simulink model "dasd"  (R2023a)
settings: Solver=VariableStepAuto  StartTime=0.0  StopTime=10.0  RelTol=1e-3
libraries: simulink x2, commdigbbndpm3 x2, commchan3 x1, commrandsrc3 x1, commsink2 x1
settings Model: Creator=aedan  LastModifiedBy=aedan

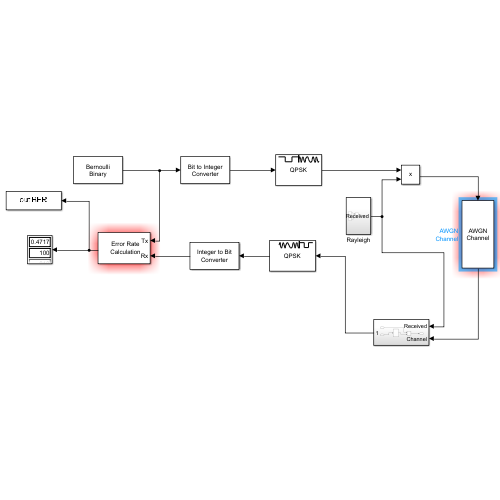
[thumbnail: Simulink's stored preview of the top-level diagram]
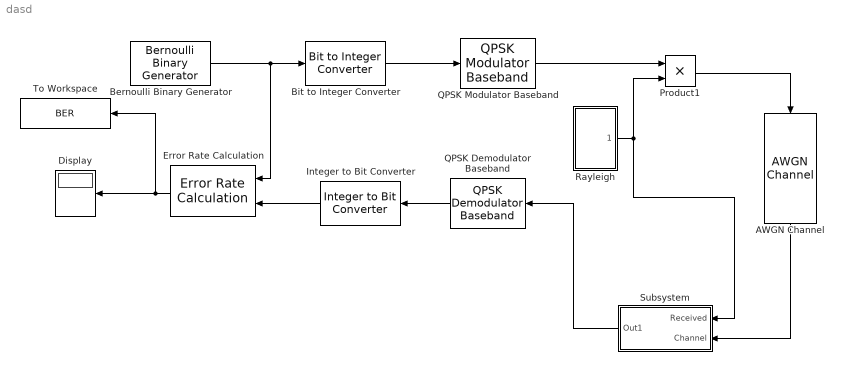
== system dasd ==
  AWGN Channel : commchan3/AWGN Channel  LegacyMode=off  NoiseMethod="Signal to noise ratio  (SNR)"  noiseMode="Signal to noise ratio  (SNR)"  EbNo=EbNo  EsNo=10  SNR=EbNo  BitsPerSymbol=1  SignalPower=1  SamplesPerSymbol=1  SymbolPeriod=1  VarianceSource=Parameter  Variance=1  RandomStream=Global stream  Seed=67  SimulateUsing=Code generation
  Bernoulli Binary Generator : commrandsrc3/Bernoulli Binary Generator  ProbabilityOfZero=0.5  SeedSource=Auto  Seed=0  SampleTime=1e-6  SamplesPerFrame=2  OutputDataType=uint8  SimulateUsing=Interpreted execution
  Bit to Integer Converter : simulink/Logic and Bit Operations/Bit to Integer Converter  nbits=2  bitOrder=MSB first  signedOutputValues=Unsigned  outDtype=Inherit via internal rule  outDtypeSigned=Inherit via internal rule
  Display : Display
  Error Rate Calculation : commsink2/Error Rate Calculation  N=0  st_delay=0  cp_mode=Entire frame  subframe=[]  PMode=Port  WsName=grayBER  RsMode2=off  stop=on  numErr=maxNumErrs  maxBits=maxNumBits
  Integer to Bit Converter : simulink/Logic and Bit Operations/Integer to Bit Converter  nbits=2  signedInputValues=Unsigned  bitOrder=MSB first  outDtype=Inherit via internal rule
      settings: LibrarySourceBlock=|
      | commutil2/Integer to Bit
      | Converter
  Product1 : Product
  QPSK Demodulator Baseband : commdigbbndpm3/QPSK Demodulator Baseband  OutType=Integer  DecType=Hard decision  VarSource=Dialog  Variance=1  Dec=Gray  Ph=pi/4  outDtype1=Inherit via internal rule  outDtype2=Inherit via internal rule  derotateFactorWordLen=16  derotateFactorDataTypeStr=Inherit: Same word length as input  derotateFactorLastDataTypeStr=Inherit: Same word length as input
      settings: LibrarySourceBlock=|
      | commhdldigbbndpm/QPSK
      | Demodulator
      | Baseband
  QPSK Modulator Baseband : commdigbbndpm3/QPSK Modulator Baseband  InType=Integer  Enc=Gray  Ph=pi/4  outDtype=double  outWordLen=16  outUDDataType=sfix(16)  outFracLenMode=Best precision  outFracLen=15  outDataTypeStr=double  outLastDataTypeStr=double
  Rayleigh : Subsystem
  Subsystem : Subsystem
  To Workspace : ToWorkspace  VariableName=BER  SampleTime=-1
      settings: MaxDataPoints=1
  wires:
  Bernoulli Binary Generator/1 -> Error Rate Calculation/1, Bit to Integer Converter/1
  Bit to Integer Converter/1 -> QPSK Modulator Baseband/1
  Integer to Bit Converter/1 -> Error Rate Calculation/2
  QPSK Modulator Baseband/1 -> Product1/1
  Product1/1 -> AWGN Channel/1
  QPSK Demodulator Baseband/1 -> Integer to Bit Converter/1
  Rayleigh/1(Received) -> Subsystem/1(Received), Product1/2
  AWGN Channel/1 -> Subsystem/2(Channel)
  Subsystem/1(Out1) -> QPSK Demodulator Baseband/1
  Error Rate Calculation/1 -> To Workspace/1, Display/1

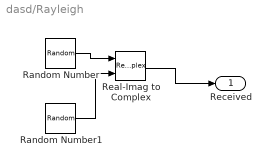
== system dasd/Rayleigh ==
  Random Number : RandomNumber  Variance=1/2  SampleTime=0.1
  Random Number1 : RandomNumber  Variance=1/2  SampleTime=0.1
  Real-Imag to Complex : RealImagToComplex
  Received : Outport
  wires:
  Random Number/1 -> Real-Imag to Complex/1
  Real-Imag to Complex/1 -> Received/1
  Random Number1/1 -> Real-Imag to Complex/2

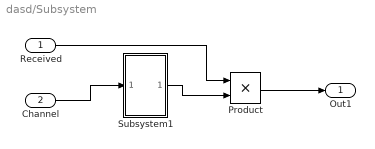
== system dasd/Subsystem ==
  Received : Inport
  Channel : Inport  Port=2
  Product : Product
  Subsystem1 : Subsystem
  Out1 : Outport
  wires:
  Product/1 -> Out1/1
  Subsystem1/1(Out1) -> Product/2
  Channel/1 -> Subsystem1/1(In1)
  Received/1 -> Product/1

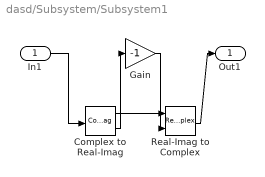
== system dasd/Subsystem/Subsystem1 ==
  In1 : Inport
  Complex to Real-Imag : ComplexToRealImag
  Gain : Gain  Gain=-1
  Real-Imag to Complex : RealImagToComplex
  Out1 : Outport
  wires:
  Complex to Real-Imag/2 -> Gain/1
  Complex to Real-Imag/1 -> Real-Imag to Complex/1
  In1/1 -> Complex to Real-Imag/1
  Real-Imag to Complex/1 -> Out1/1
  Gain/1 -> Real-Imag to Complex/2
